simulink model "NarksPrviModel3Random"  (R2017a)
settings: Solver=VariableStepAuto  StartTime=0.0  StopTime=10  RelTol=1e-3
settings Model: Creator=Korisnik  LastModifiedBy=Korisnik

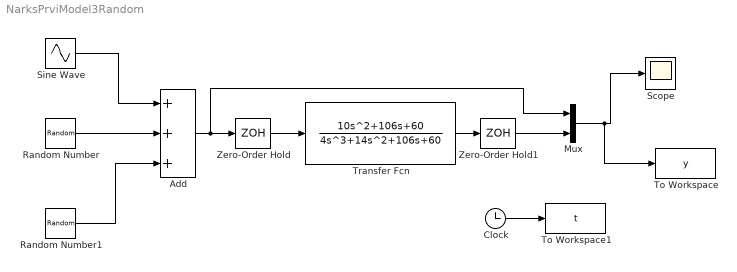
== system NarksPrviModel3Random ==
  Add : Sum  Inputs=3
  Clock : Clock
  Mux : Mux  Inputs=2
  Random Number : RandomNumber  Variance=0.1  SampleTime=0.1
  Random Number1 : RandomNumber  Variance=0.01  SampleTime=0.1
  Scope : Scope
  Sine Wave : Sin  Amplitude=5  Frequency=10  SampleTime=0.1
  To Workspace : ToWorkspace  VariableName=y  SampleTime=-1
  To Workspace1 : ToWorkspace  VariableName=t  SampleTime=-1
  Transfer Fcn : TransferFcn  Numerator=[0 10 106 60]  Denominator=[4 14 106 60]
  Zero-Order Hold : ZeroOrderHold  SampleTime=0.1
  Zero-Order Hold1 : ZeroOrderHold  SampleTime=0.1
  wires:
  Sine Wave/1 -> Add/1
  Random Number/1 -> Add/2
  Random Number1/1 -> Add/3
  Add/1 -> Mux/1, Zero-Order Hold/1
  Zero-Order Hold/1 -> Transfer Fcn/1
  Transfer Fcn/1 -> Zero-Order Hold1/1
  Zero-Order Hold1/1 -> Mux/2
  Mux/1 -> To Workspace/1, Scope/1
  Clock/1 -> To Workspace1/1
